simulink model "Car_Suspension_Model"  (R2021b)
settings: Solver=VariableStepAuto  StartTime=0.0  StopTime=2  RelTol=1e-3
values from neighbouring files (symbols this model uses):
  A = [-(b/m1) (b/m1) -(1/m1) (1/m1) ... (first row only)    [Experiment_4.m]
  B = [0;0;-Kw;0]    [Experiment_4.m]
  C = [1 0 0 0 ... (first row only)    [Experiment_4.m]
  D = [0;0]    [Experiment_4.m]
settings Model: Creator=William Watkins  LastModifiedBy=William Watkins

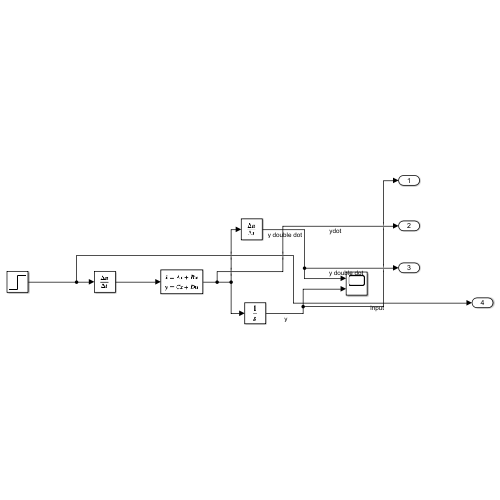
[thumbnail: Simulink's stored preview of the top-level diagram]
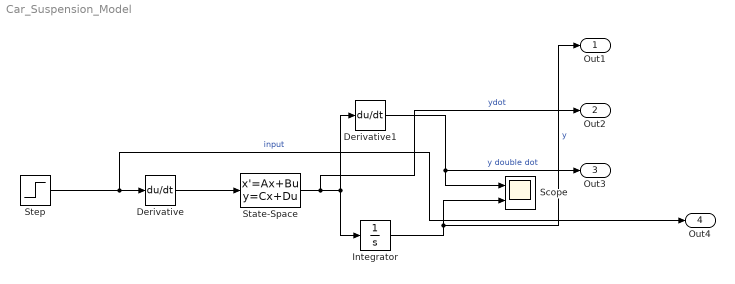
== system Car_Suspension_Model ==
  Derivative : Derivative
  Derivative1 : Derivative
  Integrator : Integrator
  Scope : Scope  NumInputPorts=2
  State-Space : StateSpace  A=A  B=B  C=C  D=D  InitialCondition=[0;0;0;0]
  Step : Step  SampleTime=0
  Out1 : Outport
  Out2 : Outport  Port=2
  Out3 : Outport  Port=3
  Out4 : Outport  Port=4
  wires:
  Step/1 -> Out4/1, Derivative/1  "input"
  Derivative/1 -> State-Space/1
  State-Space/1 -> Out2/1, Integrator/1, Derivative1/1  "ydot"
  Derivative1/1 -> Out3/1, Scope/1  "y double dot"
  Integrator/1 -> Out1/1, Scope/2  "y"
